simulink model "AIE_Kernel_Ex1"  (R2025a)
settings: Solver=VariableStepAuto  StartTime=0.0  StopTime=10.0  RelTol=1e-3
undefined symbols (not defined in the file): i, L, nsvg1369, xcvc1502
libraries: aieBasic x2, dspsrcs4 x1, vmcUtilities x1
settings Model: Creator=abehbood  LastModifiedBy=robg
settings RTWCC: GPUComputeCapability=3.5

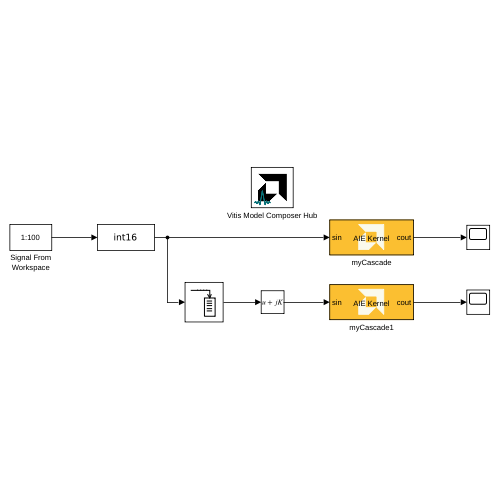
[thumbnail: Simulink's stored preview of the top-level diagram]
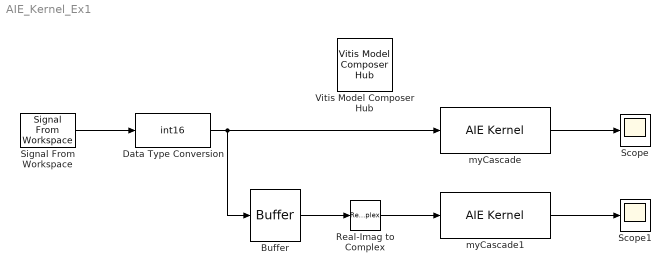
== system AIE_Kernel_Ex1 ==
  Buffer : Buffer  N=4  OutputFrames=off
  Data Type Conversion : DataTypeConversion  OutDataTypeStr=int16  SaturateOnIntegerOverflow=off  RndMeth=Floor
  Real-Imag to Complex : RealImagToComplex  Input=Real
  Scope : Scope
      settings: ActiveDisplayYMinimum=-14  ActiveDisplayYMaximum=250.8106
  Scope1 : Scope
      settings: ActiveDisplayYMinimum=-24  ActiveDisplayYMaximum=216
  Signal From Workspace : dspsrcs4/Signal From Workspace  X=1:100  Ts=1  nsamps=8  OutputAfterFinalValue=Setting to zero  ignoreOrWarnInputAndFrameLengths=off  OutputFrames=off
  Vitis Model Composer Hub : vmcUtilities/Vitis Model Composer Hub  Tag=genX  CodeGeneration=off  StartColumn=1  NumberOfColumns=1  TargetDirectory=./code  exportDesign=off  analyzeDesign=off  validateDesignOnHw=off  ExportType=AI Engines  IpVendor=xilinx.com  IpLibrary=hls  IpVersion=1.0  IpHWLanguage=Verilog  AieCompilerOptions={}  AieSimulatorOptions={}  CreateTestbench=off  TestbenchStackSize=10  RunRtlSim=off  RunCSim=off  RunAieSim=off  enableSimulationTimeout=on  enableGraphIterations=on  AieSimTimeout=50000  AieGraphIterations=-1  RunAieSimProfiling=off  LaunchVitisAnalyzer=off  PlotOutput=off  RunX86Sim=off  X86SimTimeout=10  GenHwImage=off  GenLibadfXo=off  GenHwValidationCode=off  PlatformType=Not Specified  HwSystemType=Baremetal  HwValidationTarget=hw  ProjDevice=xcvc1502-nsvg1369-1LHP-i-L  ProjDevicePart=xcvc1502-nsvg1369-1LHP-i-L  AIEType=AIE  SamplePeriod=-1  ClockFrequency=200  DataPathParallelism=1  xilinxfamily=versalaicore  part=xcvc1502  speed=-1LHP-i-L  package=nsvg1369  directory=./code  testbench=off  incr_netlist=off  synthesis_tool=Vivado  clock_wrapper=Clock Enables  dbl_ovrd=According to Block Masks  dcm_input_clock_period=10  sysclk_period=10  simulink_period=1  eval_field=0  LogFileName=''  NThreads=4
  myCascade : aieBasic/AIE Kernel  KernelAllAttrs=s[12;12;9;9;19;14;21;23;21;23;24;21;15;17;12;24;26;26;26;27;28;9;21;23;23;23;24;25;14;19;19;29]@FunctionNameDeclFileNamePortNamesPortTypesPortSerializedTypesPortDirectionsPortWindowSizeEnablesPortWindowMarginEnablesPortBufferSizeEnablesPortBufferMarginEnablesPortSynchronicityEnablesPortSignalSizeEnablesPortBufferSizesPortBufferMarginsFunctionDeclFunctionTemplateSpecKindFunctionTemplateParamNamesFunctionTemplateParamKindsFunctionTemplateParamTypesFunctionTemplateParamValuesFunctionTemplateParamEnablesClassDeclClassTemplateSpecKindClassTemplateParamNamesClassTemplateParamKindsClassTemplateParamTypesClassTemplateParamValuesClassTemplateParamEnablesClassCtorDeclsClassCtorParamNamesClassCtorParamTypesClassCtorParamSerializedTypes[1 1]@C[32 1]@t9@myCascadet17@../../myCascade.hC[2 1]@t3@sint4@coutC[2 1]@t20@input_stream_int16 *t24@output_stream< acc48 > *C[2 1]@t30@{P{Tinput_stream{1{t{Bi16}}}}}t33@{P{Toutput_stream{1{t{Sacc48}}}}}C[2 1]@t5@inputt6@outputC[2 1]@l0@l0@C[2 1]@l0@l0@C[2 1]@l0@l0@C[2 1]@l0@l0@C[2 1]@l0@l0@C[2 1]@l0@l1@C[2 1]@nnC[2 1]@nnt71@void myCascade(input_stream_int16 * sin, output_stream< acc48 > * cout)t4@nonee[0 1]@e[0 1]@e[0 1]@e[0 1]@e[0 1]@nne[0 1]@e[0 1]@e[0 1]@e[0 1]@e[0 1]@e[0 1]@e[0 1]@e[0 1]@e[0 1]@  PortNames={'sin'; 'cout'}  PortSerializedTypes={'{P{Tinput_stream{1{t{Bi16}}}}}'; '{P{Toutput_stream{1{t{Sacc48}}}}}'}  PortWindowSizes={0.000000000000000000e+00, 0.000000000000000000e+00}  PortWindowMargins={0.000000000000000000e+00, 0.000000000000000000e+00}  PortSynchronicities={'auto', 'auto'}  PortSignalSizes={0.000000000000000000e+00; 8.000000000000000000e+00}  FunctionTemplateSpecKind=none  FunctionTemplateParamNames={}  FunctionTemplateParamKinds={}  FunctionTemplateParamTypes={}  FunctionTemplateParamValues={}  FunctionIndex=1  FunctionTabVisible=on  FunctionTemplateParamsVisible=off  FunctionDeclTypeOptions=C[1 1]@t71@void myCascade(input_stream_int16 * sin, output_stream< acc48 > * cout)  FunctionDecl=void myCascade(input_stream_int16 * sin, output_stream< acc48 > * cout)  FunctionTemplateParams={}  FunctionTemplateParamsEnables={}  PortAttrs={ 'input', 'sin', 'input_stream_int16 *', '', '', '', ''; 'output', 'cout', 'output_stream< acc48 > *', '', '', '', '8' }  PortAttrsEnables={'off', 'off', 'off', 'off', 'off', 'off', 'off';'off', 'off', 'off', 'off', 'off', 'off', 'on'}  SampleTime=-1  KernelHeaderFile=myCascade.h  KernelFunction=myCascade  KernelSourceFile=myCascade.cpp  KernelSearchPaths={}  PreProcOptions={}  blockJsonConstraints=[]
  myCascade1 : aieBasic/AIE Kernel  KernelAllAttrs=s[12;12;9;9;19;14;21;23;21;23;24;21;15;17;12;24;26;26;26;27;28;9;21;23;23;23;24;25;14;19;19;29]@FunctionNameDeclFileNamePortNamesPortTypesPortSerializedTypesPortDirectionsPortWindowSizeEnablesPortWindowMarginEnablesPortBufferSizeEnablesPortBufferMarginEnablesPortSynchronicityEnablesPortSignalSizeEnablesPortBufferSizesPortBufferMarginsFunctionDeclFunctionTemplateSpecKindFunctionTemplateParamNamesFunctionTemplateParamKindsFunctionTemplateParamTypesFunctionTemplateParamValuesFunctionTemplateParamEnablesClassDeclClassTemplateSpecKindClassTemplateParamNamesClassTemplateParamKindsClassTemplateParamTypesClassTemplateParamValuesClassTemplateParamEnablesClassCtorDeclsClassCtorParamNamesClassCtorParamTypesClassCtorParamSerializedTypes[1 1]@C[32 1]@t11@myCascade_ct17@../../myCascade.hC[2 1]@t3@sint4@coutC[2 1]@t21@input_stream_cint16 *t25@output_stream< cacc48 > *C[2 1]@t33@{P{Tinput_stream{1{t{Scint16}}}}}t34@{P{Toutput_stream{1{t{Scacc48}}}}}C[2 1]@t5@inputt6@outputC[2 1]@l0@l0@C[2 1]@l0@l0@C[2 1]@l0@l0@C[2 1]@l0@l0@C[2 1]@l0@l0@C[2 1]@l0@l1@C[2 1]@nnC[2 1]@nnt75@void myCascade_c(input_stream_cint16 * sin, output_stream< cacc48 > * cout)t4@nonee[0 1]@e[0 1]@e[0 1]@e[0 1]@e[0 1]@nne[0 1]@e[0 1]@e[0 1]@e[0 1]@e[0 1]@e[0 1]@e[0 1]@e[0 1]@e[0 1]@  PortNames={'sin'; 'cout'}  PortSerializedTypes={'{P{Tinput_stream{1{t{Scint16}}}}}'; '{P{Toutput_stream{1{t{Scacc48}}}}}'}  PortWindowSizes={0.000000000000000000e+00, 0.000000000000000000e+00}  PortWindowMargins={0.000000000000000000e+00, 0.000000000000000000e+00}  PortSynchronicities={'auto', 'auto'}  PortSignalSizes={0.000000000000000000e+00; 4.000000000000000000e+00}  FunctionTemplateSpecKind=none  FunctionTemplateParamNames={}  FunctionTemplateParamKinds={}  FunctionTemplateParamTypes={}  FunctionTemplateParamValues={}  FunctionIndex=1  FunctionTabVisible=on  FunctionTemplateParamsVisible=off  FunctionDeclTypeOptions=C[1 1]@t75@void myCascade_c(input_stream_cint16 * sin, output_stream< cacc48 > * cout)  FunctionDecl=void myCascade_c(input_stream_cint16 * sin, output_stream< cacc48 > * cout)  FunctionTemplateParams={}  FunctionTemplateParamsEnables={}  PortAttrs={ 'input', 'sin', 'input_stream_cint16 *', '', '', '', ''; 'output', 'cout', 'output_stream< cacc48 > *', '', '', '', '4' }  PortAttrsEnables={'off', 'off', 'off', 'off', 'off', 'off', 'off';'off', 'off', 'off', 'off', 'off', 'off', 'on'}  SampleTime=-1  KernelHeaderFile=myCascade.h  KernelFunction=myCascade_c  KernelSourceFile=myCascade.cpp  KernelSearchPaths={}  PreProcOptions={}  blockJsonConstraints=[]
  wires:
  Signal From Workspace/1 -> Data Type Conversion/1
  Data Type Conversion/1 -> Buffer/1, myCascade/1
  myCascade/1 -> Scope/1
  Buffer/1 -> Real-Imag to Complex/1
  Real-Imag to Complex/1 -> myCascade1/1
  myCascade1/1 -> Scope1/1
